simulink model "VAB_Linear"  (R2019b)
settings: Solver=VariableStepAuto  StartTime=0.0  StopTime=t_end  FixedStep=Ts  RelTol=1e-3
undefined symbols (not defined in the file or in its folder): A_real, B_real, C_real, control_on, J_m_star, k_simulazione_continua, k_t, L, phi_p_setpoint, R, sigbuilder_block, x_0
libraries: simulink x1, cstblocks x1
settings Model: EnablePacing=on  Creator=miche  LastModifiedBy=AndreaCalegari

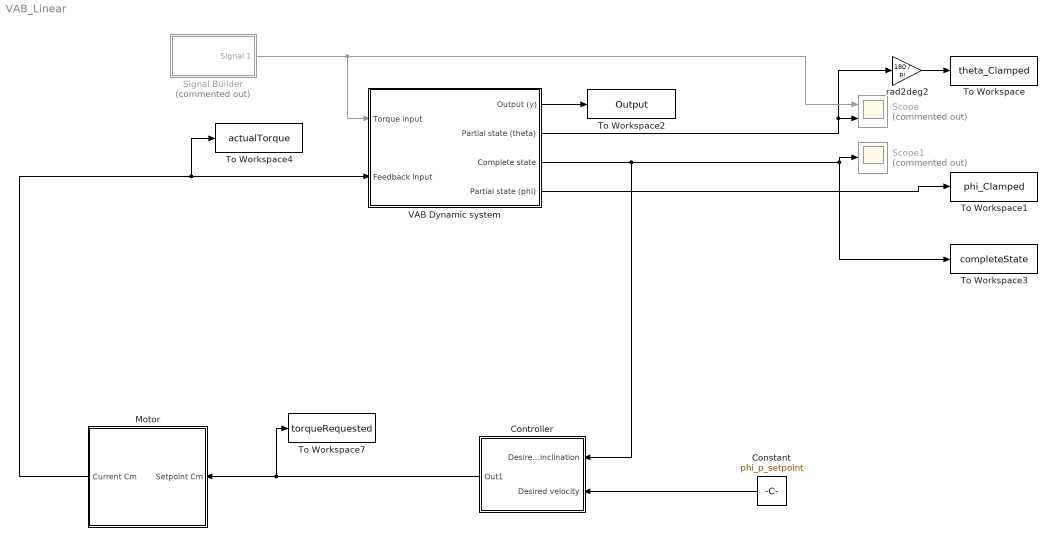
== system VAB_Linear ==
  Constant : Constant  Value=phi_p_setpoint
  Controller : Subsystem
  "Motor " : Subsystem
  Scope : Scope  Commented=on  NumInputPorts=2
  Scope1 : Scope  Commented=on
  Signal Builder : Subsystem  Tag=STV Subsys  Commented=on  LoadFcn=sigbuilder_block('load');  StartFcn=sigbuilder_block('start');  StopFcn=sigbuilder_block('stop');  ClipboardFcn=sigbuilder_block('clipboard');  mask(Sigbuilder block){tuvar=[0:10]}
      mask help: Simulink:masks:SigbuilderBlock_MD
      mask init:
      | if ~strcmp(get_param(bdroot(gcbh),'SimulationStatus'),'stopped') tuvar = sigbuilder_block('maskInit'); end
      settings: CopyFcn=sigbuilder_block('copy');  DeleteFcn=sigbuilder_block('delete');  ModelCloseFcn=sigbuilder_block('modelClose');  PreSaveFcn=sigbuilder_block('preSave');  PauseFcn=sigbuilder_block('pause');  ContinueFcn=sigbuilder_block('continue');  NameChangeFcn=sigbuilder_block('namechange');  OpenFcn=sigbuilder_block('open',[6 6 1012.5 506.25 ]);  CloseFcn=sigbuilder_block('close');
      mask Display: plot(0, 0, 100, 100,[2, 2, 32, 32, 2], [68, 8, 8, 68, 68],[32, 2], [38, 38], [32, 19, 2],[53, 60, 44], [32, 17, 17, 2],[16, 16, 31, 31]);txt = getActiveGroup(gcbh);text(2, 100, txt,'verticalAlignment', 'top');
  To Workspace : ToWorkspace  VariableName=theta_Clamped  SampleTime=-1
  To Workspace1 : ToWorkspace  VariableName=phi_Clamped  SampleTime=-1
  To Workspace2 : ToWorkspace  VariableName=Output  SampleTime=-1
  To Workspace3 : ToWorkspace  VariableName=completeState  SampleTime=-1
  To Workspace4 : ToWorkspace  VariableName=actualTorque  SampleTime=-1
  To Workspace7 : ToWorkspace  VariableName=torqueRequested  SampleTime=-1
  VAB Dynamic system : Subsystem
  rad2deg2 : Gain  Gain=180 / pi
  wires:
  VAB Dynamic system/2(Partial state (theta)) -> rad2deg2/1, Scope/2
  VAB Dynamic system/1(Output (y)) -> To Workspace2/1
  Signal Builder/1(Signal 1) -> Scope/1, VAB Dynamic system/1(Torque input)
  Constant/1 -> Controller/2("Desired velocity ")
  VAB Dynamic system/3("Complete state ") -> Controller/1(Desired inclination), To Workspace3/1, Scope1/1
  VAB Dynamic system/4(Partial state (phi)) -> To Workspace1/1
  rad2deg2/1 -> To Workspace/1
  Controller/1(Out1) -> To Workspace7/1, "Motor "/1(Setpoint Cm)
  "Motor "/1("Current Cm ") -> To Workspace4/1, VAB Dynamic system/2(Feedback input)

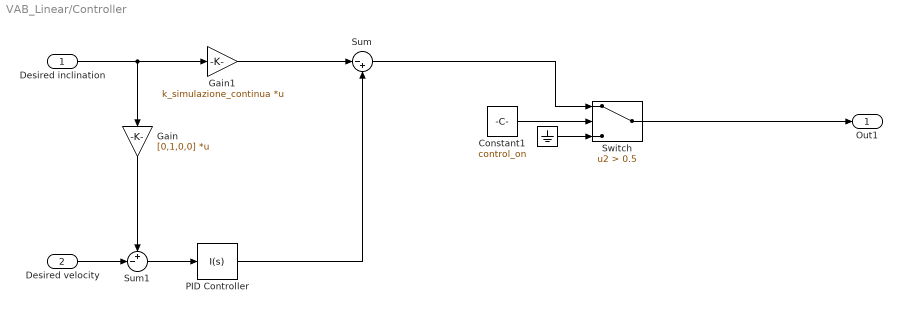
== system VAB_Linear/Controller ==
  Desired inclination : Inport
  "Desired velocity " : Inport  Port=2
  " " : Ground
  Constant1 : Constant  Value=control_on
  Gain : Gain  Gain=[0,1,0,0]  Multiplication=Matrix(K*u)
  Gain1 : Gain  Gain=k_simulazione_continua  Multiplication=Matrix(K*u)
  PID Controller : simulink/Continuous/PID Controller  Controller=I  Form=Parallel  TimeDomain=Continuous-time  SampleTime=-1  IntegratorMethod=Forward Euler  FilterMethod=Forward Euler  ControllerParametersSource=internal  P=0.0180494069153199  I=0.00227178510009537  D=0.0209925781921424  UseFilter=on  N=0.59543101805034  TunerSelectOption=Transfer Function Based (PID Tuner App)  InitialConditionSource=internal  InitialConditionForIntegrator=0  InitialConditionForFilter=0  DifferentiatorICPrevScaledInput=0  ExternalReset=none  TrackingMode=off  Kt=1  LimitOutput=off  UpperSaturationLimit=inf  LowerSaturationLimit=-inf  LinearizeAsGain=on  AntiWindupMode=none  Kb=1  POutMin=[]  POutMax=[]  IOutMin=[]  IOutMax=[]  DOutMin=[]  DOutMax=[]  NOutMin=[]  NOutMax=[]  SumOutMin=[]  SumOutMax=[]  SaturationOutMin=[]  SaturationOutMax=[]  PParamMin=[]  PParamMax=[]  IParamMin=[]  IParamMax=[]  DParamMin=[]  DParamMax=[]  NParamMin=[]  NParamMax=[]  KbParamMin=[]  KbParamMax=[]  KtParamMin=[]  KtParamMax=[]  KbOutMin=[]  KbOutMax=[]  KtOutMin=[]  KtOutMax=[]  IntegratorOutMin=[]  IntegratorOutMax=[]  FilterOutMin=[]  FilterOutMax=[]  SumI1OutMin=[]  SumI1OutMax=[]  SumI2OutMin=[]  SumI2OutMax=[]  SumI3OutMin=[]  SumI3OutMax=[]  SumI4OutMin=[]  SumI4OutMax=[]  SumDOutMin=[]  SumDOutMax=[]  DifferentiatorOutMin=[]  DifferentiatorOutMax=[]  FilterDiffOutCoefMin=[]  FilterDiffOutCoefMax=[]  ReciprocalOutMin=[]  ReciprocalOutMax=[]  SumDenOutMin=[]  SumDenOutMax=[]  SumNumOutMin=[]  SumNumOutMax=[]  DivideOutMin=[]  DivideOutMax=[]  IntegratorContinuousStateAttributes=''  IntegratorStateMustResolveToSignalObject=off  IntegratorRTWStateStorageClass=Auto  FilterContinuousStateAttributes=''  FilterStateMustResolveToSignalObject=off  FilterRTWStateStorageClass=Auto  ParallelPVariant=Disabled  IdealPVariant=Disabled  IVariant=InternalParameters  DVariant=Disabled  IntegratorVariant=Continuous  SatVariant=Disabled  AWVariant=Passthrough  PCopyVariant=Disabled  TRVariant=Disabled  FdbkBlocksVariant=Forward  IdealPFdbkVariant=Disabled  SatFdbkVariant=Disabled  DerivativeFilterVariant=Disabled  NVariant=Disabled  NCopyVariant=Disabled_SignalSpec  FilterICVariant=Disabled  IntegratorICVariant=InternalICs  ExternalResetVariant=Disabled  TRSumVariant=Passthrough  SumFdbkVariant=Disabled  SumVariant=Passthrough_I
  Sum : Sum  Inputs=|-+
  Sum1 : Sum  Inputs=+-|
  Switch : Switch  Criteria=u2 > Threshold  Threshold=0.5
  Out1 : Outport
  wires:
  Switch/1 -> Out1/1
  Constant1/1 -> Switch/2
  " "/1 -> Switch/3
  Desired inclination/1 -> Gain1/1, Gain/1
  Gain/1 -> Sum1/1
  "Desired velocity "/1 -> Sum1/2
  Sum1/1 -> PID Controller/1
  Gain1/1 -> Sum/1
  PID Controller/1 -> Sum/2
  Sum/1 -> Switch/1

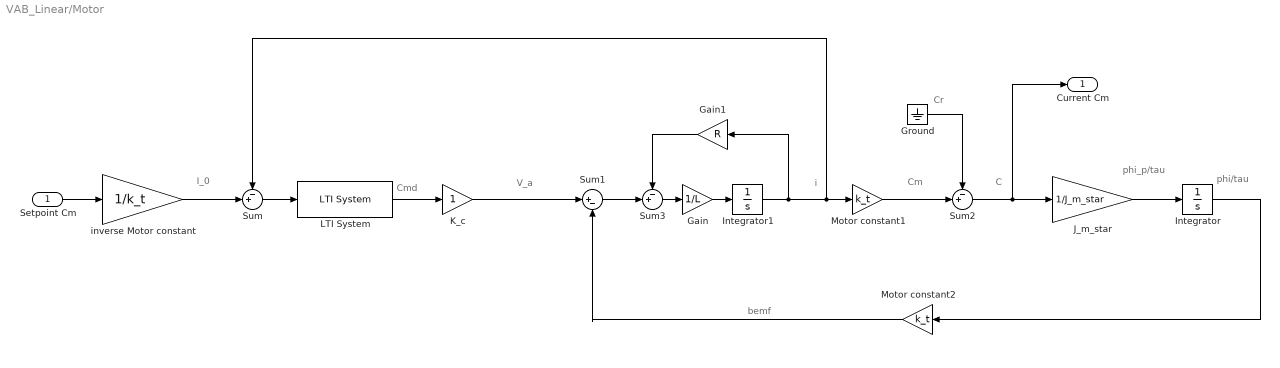
== system VAB_Linear/Motor  ==
  note: bemf
  note: phi/tau
  note: phi_p/tau
  note: C
  note: i
  note: Cmd
  note: V_a
  note: I_0
  note: Cm
  note: Cr
  Setpoint Cm : Inport
  Gain : Gain  Gain=1/L
  Gain1 : Gain  Gain=R
  Ground : Ground
  Integrator : Integrator
  Integrator1 : Integrator
  "J_m_star " : Gain  Gain=1/J_m_star
  K_c : Gain
  LTI System : cstblocks/LTI System  sys=PI_I  IC=[]
  Motor constant1 : Gain  Gain=k_t
  Motor constant2 : Gain  Gain=k_t
  Sum : Sum  Inputs=-+|
  Sum1 : Sum  Inputs=|+-
  Sum2 : Sum  Inputs=-+|
  Sum3 : Sum  Inputs=-+|
  inverse Motor constant : Gain  Gain=1/k_t
  "Current Cm " : Outport
  wires:
  Integrator/1 -> Motor constant2/1
  Motor constant1/1 -> Sum2/2
  K_c/1 -> Sum1/1
  Integrator1/1 -> Gain1/1, Sum/1, Motor constant1/1
  inverse Motor constant/1 -> Sum/2
  Sum2/1 -> "Current Cm "/1, "J_m_star "/1
  "J_m_star "/1 -> Integrator/1
  Ground/1 -> Sum2/1
  Motor constant2/1 -> Sum1/2
  Setpoint Cm/1 -> inverse Motor constant/1
  Gain/1 -> Integrator1/1
  Sum3/1 -> Gain/1
  Sum1/1 -> Sum3/2
  Gain1/1 -> Sum3/1
  Sum/1 -> LTI System/1
  LTI System/1 -> K_c/1

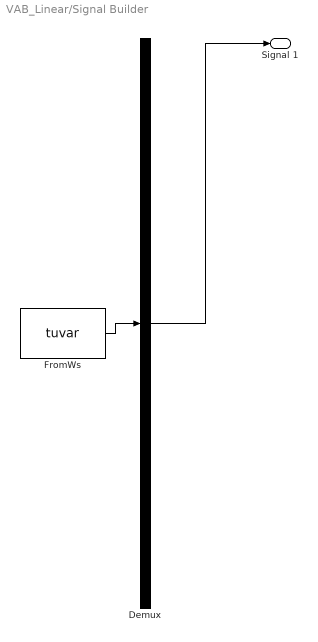
== system VAB_Linear/Signal Builder ==
  Demux : Demux  Tag=STV Demux  Outputs=1
  FromWs : FromWorkspace  Tag=STV FromWs  VariableName=tuvar  SampleTime=0
      SigBuilderData=|
      | common.afterFinalStr = 'Extrapolate'
      | common.sampleTime = 0
      | dataSet.timeRange = [0 10]
      | dataSet.name = 'Group 1'
      | sbobj.Groups.Name = 'Group 1'
      | sbobj.Groups.Signals.Name = 'Signal 1'
      | sbobj.Groups.Signals.XData = [0 4 4 4.58 4.58 10]
      | sbobj.Groups.Signals.YData = [0 0 0.998 1 0 0]
  Signal 1 : Outport  Tag=STV Outport
  wires:
  Demux/1 -> Signal 1/1
  FromWs/1 -> Demux/1

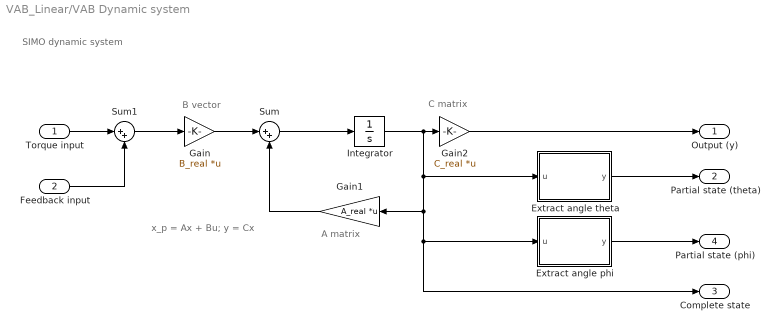
== system VAB_Linear/VAB Dynamic system ==
  note: C matrix
  note: SIMO dynamic system
  note: x_p = Ax + Bu;
      | y = Cx
  note: B vector
  note: A matrix
  Torque input : Inport
  Feedback input : Inport  Port=2
  Extract angle phi : MATLAB Function  TreatAsAtomicUnit=on
  Extract angle theta : MATLAB Function  TreatAsAtomicUnit=on
  Gain : Gain  Gain=B_real  Multiplication=Matrix(K*u) (u vector)
  Gain1 : Gain  Gain=A_real  Multiplication=Matrix(K*u) (u vector)
  Gain2 : Gain  Gain=C_real  Multiplication=Matrix(K*u) (u vector)
  Integrator : Integrator  InitialCondition=x_0
  Sum : Sum  Inputs=|++
  Sum1 : Sum  Inputs=|++
  Output (y) : Outport
  Partial state (theta) : Outport  Port=2
  "Complete state " : Outport  Port=3
  Partial state (phi) : Outport  Port=4
  wires:
  Gain2/1 -> Output (y)/1
  Gain1/1 -> Sum/2
  Gain/1 -> Sum/1
  Sum/1 -> Integrator/1
  Sum1/1 -> Gain/1
  Feedback input/1 -> Sum1/2
  Torque input/1 -> Sum1/1
  Integrator/1 -> Gain2/1, Extract angle theta/1(u), Extract angle phi/1(u), "Complete state "/1, Gain1/1
  Extract angle theta/1(y) -> Partial state (theta)/1
  Extract angle phi/1(y) -> Partial state (phi)/1

== matlab function VAB_Linear/VAB Dynamic system/Extract angle phi ==
  data: u input; y output
function y = fcn(u)

% if u(1) ~= 0
%    u(1) = mod(u(1), 2 * pi); 
% end
% 
% y = rad2deg(u(1));
y = u(1);

== matlab function VAB_Linear/VAB Dynamic system/Extract angle theta ==
  data: u input; y output
function y = fcn(u)

% if u(3) ~= 0
%    u(3) = mod(u(3), 2 * pi); 
% end
% 
% 
% y = rad2deg(u(3));
y = u(3);
